simulink library "Lib_LongPRACH"  (R2023b)
settings: Solver=VariableStepAuto  StartTime=0.0  StopTime=10.0  RelTol=1e-3
values from neighbouring files (symbols this model uses):
  prach = waveconfig.PRACH.Config    [hNRPRACHWaveformGenerator.m]
undefined symbols (not defined in the file or in its folder): AdvDSPBChannelOutDisplay, AdvDSPBDMemDisplay, AdvDSPBInDisplay, AdvDSPBOutDisplay, dpoly, dspba, dspba_ChannelInVis, dspba_ChannelOutVis, dspba_internal_get_channel_ports, evalAionMaskParam, latency, latencyCorrection, NTxAnts, primtype, UseDontCare, value
libraries: DSPBAPrim x553, DSPBABase x32, DSPBAFilters x24, DSPBAControl x18, DSPBAModelBus x8, DSPBAWaveformSynth x4, DspbAdvFftLibrary x2, DSPBAUtilities x2
(part 5 of 8)

== system Lib_LongPRACH/prach_wrap/SYM_SELECT/Zero_insertion ==
  valid_in : Inport
  chin : Inport  Port=2
  datain : Inport  Port=3
  To Workspace1 : ToWorkspace  VariableName=zeropad_front_ch  SampleTime=-1
  To Workspace2 : ToWorkspace  VariableName=zeropad_front_data  SampleTime=-1
  To Workspace7 : ToWorkspace  VariableName=zeropad_front_v  SampleTime=-1
  Zeropad_front : Subsystem
  Zeropad_rear : Subsystem
  valid_out : Outport
  "chout " : Outport  Port=2
  dataout : Outport  Port=3
  wires:
  valid_in/1 -> Zeropad_front/1(valid_in)
  datain/1 -> Zeropad_front/3(datain)
  chin/1 -> Zeropad_front/2(chin)
  Zeropad_front/1(valid_out) -> To Workspace7/1, Zeropad_rear/1(valid_in)
  Zeropad_front/2("chout ") -> To Workspace1/1, Zeropad_rear/2(chin)
  Zeropad_front/3(dataout) -> To Workspace2/1, Zeropad_rear/3(datain)
  Zeropad_rear/1(valid_out) -> valid_out/1
  Zeropad_rear/2("chout ") -> "chout "/1
  Zeropad_rear/3(dataout) -> dataout/1

== system Lib_LongPRACH/Longprach_C_M_plane/LongPRACH_core/CP_REMOVAL/RemoveCP5 ==
  vin : Inport
  chin : Inport  Port=2
  din : Inport  Port=3
  cp_start : Inport  Port=4
  gt_end : Inport  Port=5
  filt_flush_en : Inport  Port=6
  And1 : DSPBAPrim/And  primtype=and  nInputs=3  nOutputs=1  omode=Inherit via internal rule  otype=sfix(16)  scale=2^-15  rndmethod=Unbiased  factor=1  satmethod=Symmetric  shift_vec=[0 1 2 -1]  value=0  inPortNames=[' '; ' '; ' '; ' '; ' '; ' '; ' '; ' '; ' '; ' '; ' '; ' '; ' '; ' '; ' '; ' '; ]  outPortNames=[' ']  dspbaimage=dspba_prim.svg  text=fprintf('&');  style=Optimised  visibilities=8+2  version=20211007
  And2 : DSPBAPrim/And  primtype=and  nInputs=3  nOutputs=1  omode=Inherit via internal rule  otype=sfix(16)  scale=2^-15  rndmethod=Unbiased  factor=1  satmethod=Symmetric  shift_vec=[0 1 2 -1]  value=0  inPortNames=[' '; ' '; ' '; ' '; ' '; ' '; ' '; ' '; ' '; ' '; ' '; ' '; ' '; ' '; ' '; ' '; ]  outPortNames=[' ']  dspbaimage=dspba_prim.svg  text=fprintf('&');  style=Optimised  visibilities=8+2  version=20211007
  ChannelIn : DSPBAPrim/ChannelIn  primtype=channelin  nInputs=dspba_internal_get_channel_ports(gcb)  nOutputs=dspba_internal_get_channel_ports(gcb)  omode=Inherit via internal rule  otype=sfix(16)  scale=2^-15  rndmethod=Unbiased  factor=1  satmethod=Symmetric  shift_vec=[0 1 2 -1]  value=4  inPortNames=['v'; 'c'; '0'; '1'; '2'; '3'; '4'; '5'; '6'; '7'; '8'; '9'; 'A'; 'B'; 'D'; 'E'; 'F'; 'G'; 'H'; 'I'; 'J'; 'K'; 'L'; 'M'; 'N'; 'O'; 'P'; 'Q'; 'R'; 'S'; 'T'; 'U'; 'W'; 'X'; 'Y'; 'Z']  outPortNames=['v'; 'c'; '0'; '1'; '2'; '3'; '4'; '5'; '6'; '7'; '8'; '9'; 'A'; 'B'; 'D'; 'E'; 'F'; 'G'; 'H'; 'I'; 'J'; 'K'; 'L'; 'M'; 'N'; 'O'; 'P'; 'Q'; 'R'; 'S'; 'T'; 'U'; 'W'; 'X'; 'Y'; 'Z']  dspbaimage=dspba_prim_channel_tall.svg  text=fprintf('In');  style=Optimised  dataSignals=4  foldingEnabled=off  channels=1  sampleRate=200  packetBeginPresent=off  packetBeginEnabled=off  visibilities=dspba_ChannelInVis(gcb)  latencyCorrection=0  scheduleOrigin=on  version=20211214
  ChannelOut : DSPBAPrim/ChannelOut  primtype=channelout  nInputs=dspba_internal_get_channel_ports(gcb)  nOutputs=dspba_internal_get_channel_ports(gcb)  omode=Inherit via internal rule  otype=sfix(16)  scale=2^-15  rndmethod=Unbiased  factor=1  satmethod=Symmetric  shift_vec=[0 1 2 -1]  value=3  inPortNames=['v'; 'c'; '0'; '1'; '2'; '3'; '4'; '5'; '6'; '7'; '8'; '9'; 'A'; 'B'; 'D'; 'E'; 'F'; 'G'; 'H'; 'I'; 'J'; 'K'; 'L'; 'M'; 'N'; 'O'; 'P'; 'Q'; 'R'; 'S'; 'T'; 'U'; 'W'; 'X'; 'Y'; 'Z']  outPortNames=['v'; 'c'; '0'; '1'; '2'; '3'; '4'; '5'; '6'; '7'; '8'; '9'; 'A'; 'B'; 'D'; 'E'; 'F'; 'G'; 'H'; 'I'; 'J'; 'K'; 'L'; 'M'; 'N'; 'O'; 'P'; 'Q'; 'R'; 'S'; 'T'; 'U'; 'W'; 'X'; 'Y'; 'Z']  dspbaimage=dspba_prim_channel_tall.svg  text=fprintf('Out%s', AdvDSPBChannelOutDisplay(latency));  style=Optimised  dataSignals=3  foldingEnabled=off  channels=1  sampleRate=200  packetBeginPresent=off  packetBeginEnabled=off  visibilities=dspba_ChannelOutVis(gcb)  latency=3  latencyCorrection=0  version=20211214
  CmpGE_cpstart : DSPBAPrim/CmpGE  primtype=cmpgte  nInputs=2  nOutputs=1  omode=boolean  otype=sfix(16)  scale=2^-15  rndmethod=Unbiased  factor=1  satmethod=Symmetric  shift_vec=[0 1 2 -1]  value=0  inPortNames=['a'; 'b';]  outPortNames=[' ']  dspbaimage=dspba_prim.svg  text=fprintf('a>=b');  style=Optimised  visibilities=0  advOptions=[]  version=20211007
  CmpGE_cpstart1 : DSPBAPrim/CmpGE  primtype=cmpgte  nInputs=2  nOutputs=1  omode=boolean  otype=sfix(16)  scale=2^-15  rndmethod=Unbiased  factor=1  satmethod=Symmetric  shift_vec=[0 1 2 -1]  value=0  inPortNames=['a'; 'b';]  outPortNames=[' ']  dspbaimage=dspba_prim.svg  text=fprintf('a>=b');  style=Optimised  visibilities=0  advOptions=[]  version=20211007
  CmpLT_gaurdtime : DSPBAPrim/CmpLT  primtype=cmplt  nInputs=2  nOutputs=1  omode=boolean  otype=sfix(16)  scale=2^-15  rndmethod=Unbiased  factor=1  satmethod=Symmetric  shift_vec=[0 1 2 -1]  value=0  inPortNames=['a'; 'b';]  outPortNames=[' ']  dspbaimage=dspba_prim.svg  text=fprintf('a<b');  style=Optimised  visibilities=0  advOptions=[]  version=20211007
  CmpLT_gaurdtime1 : DSPBAPrim/CmpLT  primtype=cmplt  nInputs=2  nOutputs=1  omode=boolean  otype=sfix(16)  scale=2^-15  rndmethod=Unbiased  factor=1  satmethod=Symmetric  shift_vec=[0 1 2 -1]  value=0  inPortNames=['a'; 'b';]  outPortNames=[' ']  dspbaimage=dspba_prim.svg  text=fprintf('a<b');  style=Optimised  visibilities=0  advOptions=[]  version=20211007
  Const : DSPBAPrim/Const  primtype=const  nInputs=0  nOutputs=1  omode=Inherit via internal rule  otype=sfix(16)  scale=2^-15  rndmethod=Unbiased  factor=1  satmethod=Symmetric  shift_vec=[0 1 2 -1]  value=filt_flush_start  inPortNames=['+'; '+';]  outPortNames=[' ']  dspbaimage=dspba_prim.svg  text=fprintf('%s', num2str(value));  style=Optimised  visibilities=8 + 1024 + 2^18 + 2^20  floatPrecision=float32_m23  warnSaturation=on  version=20211007  SampleTime=inf
  Const1 : DSPBAPrim/Const  primtype=const  nInputs=0  nOutputs=1  omode=Inherit via internal rule  otype=sfix(16)  scale=2^-15  rndmethod=Unbiased  factor=1  satmethod=Symmetric  shift_vec=[0 1 2 -1]  value=filt_flush_end  inPortNames=['+'; '+';]  outPortNames=[' ']  dspbaimage=dspba_prim.svg  text=fprintf('%s', num2str(value));  style=Optimised  visibilities=8 + 1024 + 2^18 + 2^20  floatPrecision=float32_m23  warnSaturation=on  version=20211007  SampleTime=inf
  Convert : DSPBAPrim/Convert  primtype=convert  nInputs=1  nOutputs=1  omode=boolean  otype=sfix(16)  scale=2^-15  rndmethod=Unbiased  factor=1  satmethod=None  shift_vec=[0 1 2 -1]  value=round([0:255]/17)  inPortNames=[' '; ' ';]  outPortNames=[' '; 'c']  dspbaimage=dspba_prim_wide.svg  text=fprintf('convert');  style=Optimised  visibilities=8+64+256+2^17  clipdetect=off  floatPrecision=float32_m23  advOptions=[]  version=20211007
  Counter : DSPBAPrim/Counter  primtype=counter  nInputs=1  nOutputs=1  omode=Inherit via internal rule  otype=ufix(16)  scale=2^-0  rndmethod=Unbiased  factor=1  satmethod=Symmetric  shift_vec=[0 1 2 -1]  value=[prach.symPeriod_dec-1 prach.symPeriod_dec 1]  inPortNames=[' '; ' ';]  outPortNames=[' ']  dspbaimage=dspba_prim.svg  text=fprintf('counter\n[%d %d %d]', value(1), value(2), value(3));  style=Optimised  visibilities=8 + 1024  version=20211007
  SynthesisInfo : DSPBAPrim/SynthesisInfo  primtype=synthinfo  nInputs=0  nOutputs=0  omode=Inherit via internal rule  otype=sfix(16)  scale=2^-15  rndmethod=Truncate  factor=1  satmethod=Symmetric  shift_vec=[0 1 2 -1]  value=99  inPortNames=[' '; ' ';]  outPortNames=[' ']  dspbaimage=dspba_prim_ctrl.jpg  text=fprintf('Style=%s', style);  style=Scheduled  visibilities=2^17+2^18+2^19+2^20+2^21+2^22+2^23+2^24  constraintPair=None  constraintRelation=>  constraintLimit=6  modelRefSign=+  modelRef=''  showSchedule=off  simulationMode=Use Global Value  resetMinimization=Conditional - On for ChannelIn/Out only  version=20220106
  input2 : Scope  NumInputPorts=3
  syncgen : Subsystem
  vout : Outport  VectorParamsAs1DForOutWhenUnconnected=off
  cout : Outport  Port=2  VectorParamsAs1DForOutWhenUnconnected=off
  dout : Outport  Port=3  VectorParamsAs1DForOutWhenUnconnected=off
  filt_flush : Outport  Port=4  VectorParamsAs1DForOutWhenUnconnected=off
  sync_out : Outport  Port=5
  wires:
  ChannelIn/5 -> CmpLT_gaurdtime/2
  ChannelIn/4 -> CmpGE_cpstart/2
  cp_start/1 -> ChannelIn/4
  gt_end/1 -> ChannelIn/5
  ChannelIn/3 -> ChannelOut/3
  CmpLT_gaurdtime/1 -> And1/3
  CmpGE_cpstart/1 -> And1/2
  vin/1 -> ChannelIn/1
  chin/1 -> ChannelIn/2
  din/1 -> ChannelIn/3
  ChannelOut/3 -> dout/1
  ChannelOut/2 -> cout/1
  ChannelOut/1 -> vout/1
  ChannelIn/1 -> Counter/1, input2/1, And1/1
  ChannelIn/2 -> ChannelOut/2
  And1/1 -> input2/3, ChannelOut/1
  CmpGE_cpstart1/1 -> And2/1
  Counter/1 -> CmpLT_gaurdtime1/1, CmpGE_cpstart1/1, syncgen/1(In1), CmpGE_cpstart/1, input2/2, CmpLT_gaurdtime/1
  CmpLT_gaurdtime1/1 -> And2/2
  And2/1 -> ChannelOut/4
  ChannelOut/4 -> filt_flush/1
  ChannelIn/6 -> Convert/1
  Convert/1 -> And2/3
  Const/1 -> CmpGE_cpstart1/2
  Const1/1 -> CmpLT_gaurdtime1/2
  filt_flush_en/1 -> ChannelIn/6
  syncgen/1(q) -> ChannelOut/5
  ChannelOut/5 -> sync_out/1

== system Lib_LongPRACH/Longprach_C_M_plane/LongPRACH_core/DECIMATION1/Stage1 ==
  data_in : Inport
  valid_in : Inport  Port=2
  ch_in : Inport  Port=3
  flush_en : Inport  Port=4
  Filt_DEC_by_3_stage1 : Subsystem
  filt_flush_in : Subsystem
  data_out : Outport
  valid_out : Outport  Port=2
  ch_out : Outport  Port=3
  wires:
  Filt_DEC_by_3_stage1/3(cout) -> ch_out/1
  Filt_DEC_by_3_stage1/2(vout) -> valid_out/1
  data_in/1 -> filt_flush_in/1(data_in)
  filt_flush_in/1(data_out) -> Filt_DEC_by_3_stage1/1(din)
  Filt_DEC_by_3_stage1/1(dout) -> data_out/1
  filt_flush_in/2(valid_out) -> Filt_DEC_by_3_stage1/2(vin)
  filt_flush_in/3(ch_out) -> Filt_DEC_by_3_stage1/3(cin)
  flush_en/1 -> filt_flush_in/4(flush_en)
  valid_in/1 -> filt_flush_in/2(valid_in)
  ch_in/1 -> filt_flush_in/3(ch_in)

== system Lib_LongPRACH/Longprach_C_M_plane/LongPRACH_core/DECIMATION1/Stage2 ==
  data_in : Inport
  valid_in : Inport  Port=2
  ch_in : Inport  Port=3
  Filt_DEC_by_2_stage2 : Subsystem
  data_out : Outport
  valid_out : Outport  Port=2
  ch_out : Outport  Port=3
  wires:
  data_in/1 -> Filt_DEC_by_2_stage2/1(din)
  valid_in/1 -> Filt_DEC_by_2_stage2/2(vin)
  ch_in/1 -> Filt_DEC_by_2_stage2/3(cin)
  Filt_DEC_by_2_stage2/1(dout) -> data_out/1
  Filt_DEC_by_2_stage2/3(cout) -> ch_out/1
  Filt_DEC_by_2_stage2/2(vout) -> valid_out/1

== system Lib_LongPRACH/Longprach_C_M_plane/LongPRACH_core/DECIMATION1/Stage3 ==
  data_in : Inport
  valid_in : Inport  Port=2
  ch_in : Inport  Port=3
  Filt_DEC_by_2_stage3 : Subsystem
  data_out : Outport
  valid_out : Outport  Port=2
  ch_out : Outport  Port=3
  wires:
  valid_in/1 -> Filt_DEC_by_2_stage3/2(vin)
  Filt_DEC_by_2_stage3/1(dout) -> data_out/1
  Filt_DEC_by_2_stage3/3(cout) -> ch_out/1
  Filt_DEC_by_2_stage3/2(vout) -> valid_out/1
  ch_in/1 -> Filt_DEC_by_2_stage3/3(cin)
  data_in/1 -> Filt_DEC_by_2_stage3/1(din)

== system Lib_LongPRACH/Longprach_C_M_plane/LongPRACH_core/DECIMATION1/Stage5 ==
  data_in : Inport
  valid_in : Inport  Port=2
  ch_in : Inport  Port=3
  Filt_DEC_by_2_stage5 : Subsystem
  data_out : Outport
  valid_out : Outport  Port=2
  ch_out : Outport  Port=3
  wires:
  Filt_DEC_by_2_stage5/1(dout) -> data_out/1
  Filt_DEC_by_2_stage5/3(cout) -> ch_out/1
  data_in/1 -> Filt_DEC_by_2_stage5/1(din)
  Filt_DEC_by_2_stage5/2(vout) -> valid_out/1
  valid_in/1 -> Filt_DEC_by_2_stage5/2(vin)
  ch_in/1 -> Filt_DEC_by_2_stage5/3(cin)

== system Lib_LongPRACH/Longprach_C_M_plane/LongPRACH_core/DECIMATION1/Stage6 ==
  data_in : Inport
  valid_in : Inport  Port=2
  ch_in : Inport  Port=3
  flush_en : Inport  Port=4
  Filt_DEC_by_2_stage6 : Subsystem
  filt_flush_out : Subsystem
  data_out : Outport
  valid_out : Outport  Port=2
  ch_out : Outport  Port=3
  wires:
  data_in/1 -> Filt_DEC_by_2_stage6/1(din)
  valid_in/1 -> Filt_DEC_by_2_stage6/2(vin)
  ch_in/1 -> Filt_DEC_by_2_stage6/3(cin)
  filt_flush_out/1(data_out) -> data_out/1
  filt_flush_out/2(valid_out) -> valid_out/1
  filt_flush_out/3(ch_out) -> ch_out/1
  Filt_DEC_by_2_stage6/1(dout) -> filt_flush_out/1(data_in)
  Filt_DEC_by_2_stage6/2(vout) -> filt_flush_out/2(valid_in)
  Filt_DEC_by_2_stage6/3(cout) -> filt_flush_out/3(ch_in)
  flush_en/1 -> filt_flush_out/4(flush_en)

== system Lib_LongPRACH/Longprach_C_M_plane/LongPRACH_core/DECIMATION1/stage4 ==
  data_in : Inport
  valid_in : Inport  Port=2
  ch_in : Inport  Port=3
  Filt_DEC_by_2_stage4 : Subsystem
  data_out : Outport
  valid_out : Outport  Port=2
  ch_out : Outport  Port=3
  wires:
  Filt_DEC_by_2_stage4/3(cout) -> ch_out/1
  Filt_DEC_by_2_stage4/2(vout) -> valid_out/1
  data_in/1 -> Filt_DEC_by_2_stage4/1(din)
  ch_in/1 -> Filt_DEC_by_2_stage4/3(cin)
  Filt_DEC_by_2_stage4/1(dout) -> data_out/1
  valid_in/1 -> Filt_DEC_by_2_stage4/2(vin)

== system Lib_LongPRACH/Longprach_C_M_plane/LongPRACH_core/FFTShift/ChNoLatch ==
  valid1 : Inport
  din : Inport  Port=2
  valid2 : Inport  Port=3
  FIFO : DSPBAPrim/FIFO  primtype=fifo  nInputs=3  nOutputs=4  omode=Inherit via internal rule  otype=sfix(16)  scale=2^-15  rndmethod=Unbiased  factor=1  satmethod=Symmetric  shift_vec=[0 1 2 -1]  value=[32 4 16]  inPortNames=['w'; 'd'; 'r'; 'f']  outPortNames=['v'; 'q'; 't'; 'f']  dspbaimage=dspba_prim_tall.svg  text=fprintf('fifo');  style=Optimised  visibilities=263168  version=20211007  user_sclr=off
  Terminator1 : Terminator
  Terminator2 : Terminator
  Terminator3 : Terminator
  risingedge : Subsystem
  risingedge1 : Subsystem
  dout : Outport
  wires:
  din/1 -> FIFO/2
  valid1/1 -> risingedge/1(In2)
  FIFO/2 -> dout/1
  valid2/1 -> risingedge1/1(In2)
  risingedge/1(Out1) -> FIFO/1
  FIFO/4 -> Terminator2/1
  risingedge1/1(Out1) -> FIFO/3
  FIFO/1 -> Terminator3/1
  FIFO/3 -> Terminator1/1

== system Lib_LongPRACH/Longprach_C_M_plane/LongPRACH_core/FFTShift/Mem_rd_wr ==
  valid : Inport
  Mem_rd_control : Subsystem
  Mem_wr_control : Subsystem
  Wr_addr_final : Outport
  We : Outport  Port=2
  rd_addr_final : Outport  Port=3
  rd_validout : Outport  Port=4
  wba : Outport  Port=5
  wires:
  Mem_rd_control/2(validout) -> rd_validout/1
  Mem_rd_control/1(rd_addr_final) -> rd_addr_final/1
  Mem_wr_control/3(wba) -> Mem_rd_control/1(wba), wba/1
  Mem_wr_control/2(we) -> We/1
  Mem_wr_control/1(wr_addr_final) -> Wr_addr_final/1
  valid/1 -> Mem_wr_control/1(valid)

== system Lib_LongPRACH/Longprach_C_M_plane/LongPRACH_core/FFTShift/Subsystem ==
  toggleline : Inport
  d : Inport  Port=2
  SampleDelay : DSPBAPrim/SampleDelay  primtype=sampdelay  nInputs=1  nOutputs=1  omode=Inherit via internal rule  otype=sfix(16)  scale=2^-15  rndmethod=Unbiased  factor=1  satmethod=Symmetric  shift_vec=[0 1 2 -1]  floatPrecision=float32_m23  value=1  inPortNames=[' '; ' ';]  outPortNames=[' ']  dspbaimage=dspba_prim.svg  text=dpoly(1, eye(1,value+1), 'z')  style=Optimised  visibilities=8 + 2^11 + 2^18 + 2^19  flexible=off  slackgroup=0  augmented=0  version=20211007  advOptions=[]
  Xor : DSPBAPrim/Xor  primtype=xor  nInputs=2  nOutputs=1  omode=Inherit via internal rule  otype=sfix(16)  scale=2^-15  rndmethod=Unbiased  factor=1  satmethod=Symmetric  shift_vec=[0 1 2 -1]  value=0  inPortNames=[' '; ' '; ' '; ' '; ' '; ' '; ' '; ' '; ' '; ' '; ' '; ' '; ' '; ' '; ' '; ' '; ]  outPortNames=[' ']  dspbaimage=dspba_prim.svg  text=fprintf('^');  style=Optimised  visibilities=8+2  version=20211007
  latch_0L : DSPBAControl/latch_0L
  q : Outport
  wires:
  toggleline/1 -> Xor/2, SampleDelay/1
  d/1 -> latch_0L/2
  latch_0L/1 -> q/1
  Xor/1 -> latch_0L/1
  SampleDelay/1 -> Xor/1

== system Lib_LongPRACH/Longprach_C_M_plane/LongPRACH_core/S2B_FFT/S2B ==
  data_in : Inport
  data_valid : Inport  Port=2
  chin : Inport  Port=3
  resetin : Inport  Port=4
  ChannelIn : DSPBAPrim/ChannelIn  primtype=channelin  nInputs=dspba_internal_get_channel_ports(gcb)  nOutputs=dspba_internal_get_channel_ports(gcb)  omode=Inherit via internal rule  otype=sfix(16)  scale=2^-15  rndmethod=Unbiased  factor=1  satmethod=Symmetric  shift_vec=[0 1 2 -1]  value=2  inPortNames=['v'; 'c'; '0'; '1'; '2'; '3'; '4'; '5'; '6'; '7'; '8'; '9'; 'A'; 'B'; 'D'; 'E'; 'F'; 'G'; 'H'; 'I'; 'J'; 'K'; 'L'; 'M'; 'N'; 'O'; 'P'; 'Q'; 'R'; 'S'; 'T'; 'U'; 'W'; 'X'; 'Y'; 'Z']  outPortNames=['v'; 'c'; '0'; '1'; '2'; '3'; '4'; '5'; '6'; '7'; '8'; '9'; 'A'; 'B'; 'D'; 'E'; 'F'; 'G'; 'H'; 'I'; 'J'; 'K'; 'L'; 'M'; 'N'; 'O'; 'P'; 'Q'; 'R'; 'S'; 'T'; 'U'; 'W'; 'X'; 'Y'; 'Z']  dspbaimage=dspba_prim_channel_tall.svg  text=fprintf('In');  style=Optimised  dataSignals=2  foldingEnabled=off  channels=1  sampleRate=200  packetBeginPresent=off  packetBeginEnabled=off  visibilities=dspba_ChannelInVis(gcb)  latencyCorrection=0  scheduleOrigin=on  version=20211214
  ChannelOut : DSPBAPrim/ChannelOut  primtype=channelout  nInputs=dspba_internal_get_channel_ports(gcb)  nOutputs=dspba_internal_get_channel_ports(gcb)  omode=Inherit via internal rule  otype=sfix(16)  scale=2^-15  rndmethod=Unbiased  factor=1  satmethod=Symmetric  shift_vec=[0 1 2 -1]  value=1  inPortNames=['v'; 'c'; '0'; '1'; '2'; '3'; '4'; '5'; '6'; '7'; '8'; '9'; 'A'; 'B'; 'D'; 'E'; 'F'; 'G'; 'H'; 'I'; 'J'; 'K'; 'L'; 'M'; 'N'; 'O'; 'P'; 'Q'; 'R'; 'S'; 'T'; 'U'; 'W'; 'X'; 'Y'; 'Z']  outPortNames=['v'; 'c'; '0'; '1'; '2'; '3'; '4'; '5'; '6'; '7'; '8'; '9'; 'A'; 'B'; 'D'; 'E'; 'F'; 'G'; 'H'; 'I'; 'J'; 'K'; 'L'; 'M'; 'N'; 'O'; 'P'; 'Q'; 'R'; 'S'; 'T'; 'U'; 'W'; 'X'; 'Y'; 'Z']  dspbaimage=dspba_prim_channel_tall.svg  text=fprintf('Out%s', AdvDSPBChannelOutDisplay(latency));  style=Optimised  dataSignals=1  foldingEnabled=off  channels=1  sampleRate=200  packetBeginPresent=off  packetBeginEnabled=off  visibilities=dspba_ChannelOutVis(gcb)  latency=6  latencyCorrection=0  version=20211214
  DualMem : DSPBAPrim/DualMem  primtype=dualmem  nInputs=4  nOutputs=2  omode=Inherit via internal rule  otype=sfix(16)  scale=2^-15  rndmethod=Unbiased  factor=1  satmethod=Symmetric  shift_vec=[0 1 2 -1]  value=[zeros(1024*4*2, 1)]  inPortNames=['d1'; 'a1'; 'w1'; 'd2'; 'a2'; 'w2']  outPortNames=['q1'; 'q2']  dspbaimage=dspba_prim_tall.svg  text=fprintf('dmem%s',AdvDSPBDMemDisplay(UseDontCare));  style=Optimised  visibilities=8 + 1024 + 2^17 + 2^18  UseDontCare=on  TwinWritePorts=off  init=on  ProvideReadAccess=off  version=20211007
  S2B_control : Subsystem
  SynthesisInfo : DSPBAPrim/SynthesisInfo  primtype=synthinfo  nInputs=0  nOutputs=0  omode=Inherit via internal rule  otype=sfix(16)  scale=2^-15  rndmethod=Truncate  factor=1  satmethod=Symmetric  shift_vec=[0 1 2 -1]  value=99  inPortNames=[' '; ' ';]  outPortNames=[' ']  dspbaimage=dspba_prim_ctrl.jpg  text=fprintf('Style=%s', style);  style=Scheduled  visibilities=2^17+2^18+2^19+2^20+2^21+2^22+2^23+2^24  constraintPair=None  constraintRelation=>  constraintLimit=2  modelRefSign=+  modelRef=''  showSchedule=off  simulationMode=Use Global Value  resetMinimization=Conditional - On for ChannelIn/Out only  version=20220106
  Terminator : Terminator
  Terminator1 : Terminator
  data_out : Outport
  valid_out : Outport  Port=2
  ch_no : Outport  Port=3
  wires:
  ChannelOut/2 -> ch_no/1
  S2B_control/4(rd_validout) -> ChannelOut/1
  ChannelOut/1 -> valid_out/1
  DualMem/2 -> ChannelOut/3
  ChannelOut/3 -> data_out/1
  ChannelIn/2 -> Terminator1/1, S2B_control/2(ch_no_in)
  chin/1 -> ChannelIn/2
  data_valid/1 -> ChannelIn/1
  ChannelIn/1 -> S2B_control/1(valid)
  data_in/1 -> ChannelIn/3
  ChannelIn/3 -> DualMem/1
  S2B_control/5(ch_no) -> ChannelOut/2
  S2B_control/3(rd_addr_final) -> DualMem/4
  DualMem/1 -> Terminator/1
  S2B_control/1(Wr_addr_final) -> DualMem/2
  S2B_control/2(We) -> DualMem/3
  ChannelIn/4 -> S2B_control/3(resetin)
  resetin/1 -> ChannelIn/4

== system Lib_LongPRACH/Longprach_C_M_plane/LongPRACH_core/S2B_FFT/gain ==
  data_in : Inport
  data_valid : Inport  Port=2
  chin : Inport  Port=3
  gain : Inport  Port=4
  ChannelIn : DSPBAPrim/ChannelIn  primtype=channelin  nInputs=dspba_internal_get_channel_ports(gcb)  nOutputs=dspba_internal_get_channel_ports(gcb)  omode=Inherit via internal rule  otype=sfix(16)  scale=2^-15  rndmethod=Unbiased  factor=1  satmethod=Symmetric  shift_vec=[0 1 2 -1]  value=2  inPortNames=['v'; 'c'; '0'; '1'; '2'; '3'; '4'; '5'; '6'; '7'; '8'; '9'; 'A'; 'B'; 'D'; 'E'; 'F'; 'G'; 'H'; 'I'; 'J'; 'K'; 'L'; 'M'; 'N'; 'O'; 'P'; 'Q'; 'R'; 'S'; 'T'; 'U'; 'W'; 'X'; 'Y'; 'Z']  outPortNames=['v'; 'c'; '0'; '1'; '2'; '3'; '4'; '5'; '6'; '7'; '8'; '9'; 'A'; 'B'; 'D'; 'E'; 'F'; 'G'; 'H'; 'I'; 'J'; 'K'; 'L'; 'M'; 'N'; 'O'; 'P'; 'Q'; 'R'; 'S'; 'T'; 'U'; 'W'; 'X'; 'Y'; 'Z']  dspbaimage=dspba_prim_channel_tall.svg  text=fprintf('In');  style=Optimised  dataSignals=2  foldingEnabled=off  channels=1  sampleRate=200  packetBeginPresent=off  packetBeginEnabled=off  visibilities=dspba_ChannelInVis(gcb)  latencyCorrection=0  scheduleOrigin=on  version=20211214
  ChannelOut : DSPBAPrim/ChannelOut  primtype=channelout  nInputs=dspba_internal_get_channel_ports(gcb)  nOutputs=dspba_internal_get_channel_ports(gcb)  omode=Inherit via internal rule  otype=sfix(16)  scale=2^-15  rndmethod=Unbiased  factor=1  satmethod=Symmetric  shift_vec=[0 1 2 -1]  value=1  inPortNames=['v'; 'c'; '0'; '1'; '2'; '3'; '4'; '5'; '6'; '7'; '8'; '9'; 'A'; 'B'; 'D'; 'E'; 'F'; 'G'; 'H'; 'I'; 'J'; 'K'; 'L'; 'M'; 'N'; 'O'; 'P'; 'Q'; 'R'; 'S'; 'T'; 'U'; 'W'; 'X'; 'Y'; 'Z']  outPortNames=['v'; 'c'; '0'; '1'; '2'; '3'; '4'; '5'; '6'; '7'; '8'; '9'; 'A'; 'B'; 'D'; 'E'; 'F'; 'G'; 'H'; 'I'; 'J'; 'K'; 'L'; 'M'; 'N'; 'O'; 'P'; 'Q'; 'R'; 'S'; 'T'; 'U'; 'W'; 'X'; 'Y'; 'Z']  dspbaimage=dspba_prim_channel_tall.svg  text=fprintf('Out%s', AdvDSPBChannelOutDisplay(latency));  style=Optimised  dataSignals=1  foldingEnabled=off  channels=1  sampleRate=200  packetBeginPresent=off  packetBeginEnabled=off  visibilities=dspba_ChannelOutVis(gcb)  latency=6  latencyCorrection=0  version=20211214
  Convert : DSPBAPrim/Convert  primtype=convert  nInputs=1  nOutputs=1  omode=Specify via dialog  otype=sfix(16)  scale=2^-gain_out_frac  rndmethod=Unbiased  factor=1  satmethod=None  shift_vec=[0 1 2 -1]  value=round([0:255]/17)  inPortNames=[' '; ' ';]  outPortNames=[' '; 'c']  dspbaimage=dspba_prim_wide.svg  text=fprintf('convert');  style=Optimised  visibilities=8+64+256+2^17  clipdetect=off  floatPrecision=float32_m23  advOptions=[]  version=20211007
  Mult : DSPBAPrim/Mult  primtype=mult  nInputs=2  nOutputs=1  omode=Inherit via internal rule  otype=sfix(16)  scale=2^-15  rndmethod=Unbiased  factor=1  satmethod=Symmetric  shift_vec=[0 1 2 -1]  value=0  inPortNames=[' '; ' ';]  outPortNames=[' ']  dspbaimage=dspba_prim.svg  text=fprintf('X');  style=Optimised  visibilities=8+2^18+2^19  floatPrecision=float32_m23  floatRounding=correct  advOptions=[]  version=20211007
  SynthesisInfo : DSPBAPrim/SynthesisInfo  primtype=synthinfo  nInputs=0  nOutputs=0  omode=Inherit via internal rule  otype=sfix(16)  scale=2^-15  rndmethod=Truncate  factor=1  satmethod=Symmetric  shift_vec=[0 1 2 -1]  value=99  inPortNames=[' '; ' ';]  outPortNames=[' ']  dspbaimage=dspba_prim_ctrl.jpg  text=fprintf('Style=%s', style);  style=Scheduled  visibilities=2^17+2^18+2^19+2^20+2^21+2^22+2^23+2^24  constraintPair=None  constraintRelation=>  constraintLimit=2  modelRefSign=+  modelRef=''  showSchedule=off  simulationMode=Use Global Value  resetMinimization=Conditional - On for ChannelIn/Out only  version=20220106
  data_out : Outport
  valid_out : Outport  Port=2
  ch_no : Outport  Port=3
  wires:
  ChannelOut/2 -> ch_no/1
  ChannelOut/1 -> valid_out/1
  ChannelOut/3 -> data_out/1
  ChannelIn/2 -> ChannelOut/2
  chin/1 -> ChannelIn/2
  data_valid/1 -> ChannelIn/1
  data_in/1 -> ChannelIn/3
  gain/1 -> ChannelIn/4
  ChannelIn/1 -> ChannelOut/1
  ChannelIn/3 -> Mult/1
  ChannelIn/4 -> Mult/2
  Mult/1 -> Convert/1
  Convert/1 -> ChannelOut/3

== system Lib_LongPRACH/Longprach_C_M_plane/LongPRACH_core/SYM_SELECT/Zero_insertion ==
  valid_in : Inport
  chin : Inport  Port=2
  datain : Inport  Port=3
  To Workspace1 : ToWorkspace  VariableName=zeropad_front_ch  SampleTime=-1
  To Workspace2 : ToWorkspace  VariableName=zeropad_front_data  SampleTime=-1
  To Workspace7 : ToWorkspace  VariableName=zeropad_front_v  SampleTime=-1
  Zeropad_front : Subsystem
  Zeropad_rear : Subsystem
  valid_out : Outport
  "chout " : Outport  Port=2
  dataout : Outport  Port=3
  wires:
  Zeropad_rear/3(dataout) -> dataout/1
  Zeropad_rear/2("chout ") -> "chout "/1
  Zeropad_rear/1(valid_out) -> valid_out/1
  Zeropad_front/3(dataout) -> Zeropad_rear/3(datain), To Workspace2/1
  Zeropad_front/2("chout ") -> Zeropad_rear/2(chin), To Workspace1/1
  Zeropad_front/1(valid_out) -> Zeropad_rear/1(valid_in), To Workspace7/1
  chin/1 -> Zeropad_front/2(chin)
  datain/1 -> Zeropad_front/3(datain)
  valid_in/1 -> Zeropad_front/1(valid_in)

== system Lib_LongPRACH/Longprach_C_M_plane/LongPRACH_core/Timeref_capture_fifo/rising_edge ==
  In1 : Inport
  And : DSPBAPrim/And  primtype=and  nInputs=2  nOutputs=1  omode=Inherit via internal rule  otype=sfix(16)  scale=2^-15  rndmethod=Unbiased  factor=1  satmethod=Symmetric  shift_vec=[0 1 2 -1]  value=0  inPortNames=[' '; ' '; ' '; ' '; ' '; ' '; ' '; ' '; ' '; ' '; ' '; ' '; ' '; ' '; ' '; ' '; ]  outPortNames=[' ']  dspbaimage=dspba_prim.svg  text=fprintf('&');  style=Optimised  visibilities=8+2  version=20211007
  Not : DSPBAPrim/Not  primtype=not  nInputs=1  nOutputs=1  omode=Inherit via internal rule  otype=sfix(16)  scale=2^-15  rndmethod=Unbiased  factor=1  satmethod=Symmetric  shift_vec=[0 1 2 -1]  value=0  inPortNames=[' '; ' ';]  outPortNames=[' ']  dspbaimage=dspba_prim.svg  text=fprintf('~');  style=Optimised  visibilities=8  version=20211007
  SampleDelay : DSPBAPrim/SampleDelay  primtype=sampdelay  nInputs=1  nOutputs=1  omode=Inherit via internal rule  otype=sfix(16)  scale=2^-15  rndmethod=Unbiased  factor=1  satmethod=Symmetric  shift_vec=[0 1 2 -1]  floatPrecision=float32_m23  value=1  inPortNames=[' '; ' ';]  outPortNames=[' ']  dspbaimage=dspba_prim.svg  text=dpoly(1, eye(1,value+1), 'z')  style=Optimised  visibilities=8 + 2^11 + 2^18 + 2^19  flexible=off  slackgroup=0  augmented=0  version=20211007  advOptions=[]
  Out1 : Outport
  wires:
  In1/1 -> And/1, SampleDelay/1
  SampleDelay/1 -> Not/1
  And/1 -> Out1/1
  Not/1 -> And/2

== system Lib_LongPRACH/Longprach_C_M_plane/LongPRACH_core/Timeref_capture_fifo/rising_edge1 ==
  In1 : Inport
  And : DSPBAPrim/And  primtype=and  nInputs=2  nOutputs=1  omode=Inherit via internal rule  otype=sfix(16)  scale=2^-15  rndmethod=Unbiased  factor=1  satmethod=Symmetric  shift_vec=[0 1 2 -1]  value=0  inPortNames=[' '; ' '; ' '; ' '; ' '; ' '; ' '; ' '; ' '; ' '; ' '; ' '; ' '; ' '; ' '; ' '; ]  outPortNames=[' ']  dspbaimage=dspba_prim.svg  text=fprintf('&');  style=Optimised  visibilities=8+2  version=20211007
  Not : DSPBAPrim/Not  primtype=not  nInputs=1  nOutputs=1  omode=Inherit via internal rule  otype=sfix(16)  scale=2^-15  rndmethod=Unbiased  factor=1  satmethod=Symmetric  shift_vec=[0 1 2 -1]  value=0  inPortNames=[' '; ' ';]  outPortNames=[' ']  dspbaimage=dspba_prim.svg  text=fprintf('~');  style=Optimised  visibilities=8  version=20211007
  SampleDelay : DSPBAPrim/SampleDelay  primtype=sampdelay  nInputs=1  nOutputs=1  omode=Inherit via internal rule  otype=sfix(16)  scale=2^-15  rndmethod=Unbiased  factor=1  satmethod=Symmetric  shift_vec=[0 1 2 -1]  floatPrecision=float32_m23  value=1  inPortNames=[' '; ' ';]  outPortNames=[' ']  dspbaimage=dspba_prim.svg  text=dpoly(1, eye(1,value+1), 'z')  style=Optimised  visibilities=8 + 2^11 + 2^18 + 2^19  flexible=off  slackgroup=0  augmented=0  version=20211007  advOptions=[]
  Out1 : Outport
  wires:
  In1/1 -> And/1, SampleDelay/1
  SampleDelay/1 -> Not/1
  And/1 -> Out1/1
  Not/1 -> And/2

== system Lib_LongPRACH/Longprach_C_M_plane/MUX_ConfigId/DelayValid/Delayed_valid_gen ==
  Validin : Inport
  SubFN_Change : Inport  Port=2
  start_sym : Inport  Port=3
  CmpEQ4 : DSPBAPrim/CmpEQ  primtype=cmpeq  nInputs=2  nOutputs=1  omode=boolean  otype=sfix(16)  scale=2^-15  rndmethod=Unbiased  factor=1  satmethod=Symmetric  shift_vec=[0 1 2 -1]  value=0  inPortNames=[' '; ' ';]  outPortNames=[' ']  dspbaimage=dspba_prim.svg  text=fprintf('==');  style=Optimised  visibilities=0  advOptions=[]  version=20211007
  Const3 : DSPBAPrim/Const  primtype=const  nInputs=0  nOutputs=1  omode=boolean  otype=sfix(16)  scale=2^-15  rndmethod=Unbiased  factor=1  satmethod=Symmetric  shift_vec=[0 1 2 -1]  value=1  inPortNames=['+'; '+';]  outPortNames=[' ']  dspbaimage=dspba_prim.svg  text=fprintf('%s', num2str(value));  style=Optimised  visibilities=8 + 1024 + 2^18 + 2^20  floatPrecision=float32_m23  warnSaturation=on  version=20211007  SampleTime=inf
  Const4 : DSPBAPrim/Const  primtype=const  nInputs=0  nOutputs=1  omode=Inherit via internal rule  otype=sfix(16)  scale=2^-15  rndmethod=Unbiased  factor=1  satmethod=Symmetric  shift_vec=[0 1 2 -1]  value=Delay_Valid_by  inPortNames=['+'; '+';]  outPortNames=[' ']  dspbaimage=dspba_prim.svg  text=fprintf('%s', num2str(value));  style=Optimised  visibilities=8 + 1024 + 2^18 + 2^20  floatPrecision=float32_m23  warnSaturation=on  version=20211007  SampleTime=inf
  Const5 : DSPBAPrim/Const  primtype=const  nInputs=0  nOutputs=1  omode=Inherit via internal rule  otype=sfix(16)  scale=2^-15  rndmethod=Unbiased  factor=1  satmethod=Symmetric  shift_vec=[0 1 2 -1]  value=Delayed_Valid_len  inPortNames=['+'; '+';]  outPortNames=[' ']  dspbaimage=dspba_prim.svg  text=fprintf('%s', num2str(value));  style=Optimised  visibilities=8 + 1024 + 2^18 + 2^20  floatPrecision=float32_m23  warnSaturation=on  version=20211007  SampleTime=inf
  Const6 : DSPBAPrim/Const  primtype=const  nInputs=0  nOutputs=1  omode=Inherit via internal rule  otype=sfix(16)  scale=2^-15  rndmethod=Unbiased  factor=1  satmethod=Symmetric  shift_vec=[0 1 2 -1]  value=8  inPortNames=['+'; '+';]  outPortNames=[' ']  dspbaimage=dspba_prim.svg  text=fprintf('%s', num2str(value));  style=Optimised  visibilities=8 + 1024 + 2^18 + 2^20  floatPrecision=float32_m23  warnSaturation=on  version=20211007  SampleTime=inf
  Loop : DSPBAPrim/Loop  primtype=loop  nInputs=3  nOutputs=4  omode=Inherit via internal rule  otype=sfix(16)  scale=2^-15  rndmethod=Unbiased  factor=1  satmethod=Symmetric  shift_vec=[0 1 2 -1]  value=[zeros(16, 1)]  inPortNames=['g'; 'c'; 'e']  outPortNames=['v'; 'q'; 'f'; 'l']  dspbaimage=dspba_prim_tall.svg  text=fprintf('loop');  style=Optimised  visibilities=0  version=20211007
  Loop1 : DSPBAPrim/Loop  primtype=loop  nInputs=3  nOutputs=4  omode=Inherit via internal rule  otype=sfix(16)  scale=2^-15  rndmethod=Unbiased  factor=1  satmethod=Symmetric  shift_vec=[0 1 2 -1]  value=[zeros(16, 1)]  inPortNames=['g'; 'c'; 'e']  outPortNames=['v'; 'q'; 'f'; 'l']  dspbaimage=dspba_prim_tall.svg  text=fprintf('loop');  style=Optimised  visibilities=0  version=20211007
  Mux : DSPBAPrim/Mux  primtype=mux  nInputs=evalAionMaskParam(gcb,'value',1)+1  nOutputs=1  omode=Inherit via internal rule  otype=sfix(16)  scale=2^-15  rndmethod=Unbiased  factor=1  satmethod=Symmetric  shift_vec=[0 1 2 -1]  value=2  inPortNames=['s '; 'd0'; 'd1'; 'd2'; 'd3'; 'd4'; 'd5'; 'd6'; 'd7'; 'd8'; 'd9';]  outPortNames=[' ']  dspbaimage=dspba_prim_tall.svg  text=fprintf('%s', primtype);  style=Optimised  visibilities=1032  version=20211007
  SampleDelay : DSPBAPrim/SampleDelay  primtype=sampdelay  nInputs=1  nOutputs=1  omode=Inherit via internal rule  otype=sfix(16)  scale=2^-15  rndmethod=Unbiased  factor=1  satmethod=Symmetric  shift_vec=[0 1 2 -1]  floatPrecision=float32_m23  value=1  inPortNames=[' '; ' ';]  outPortNames=[' ']  dspbaimage=dspba_prim.svg  text=dpoly(1, eye(1,value+1), 'z')  style=Optimised  visibilities=8 + 2^11 + 2^18 + 2^19  flexible=off  slackgroup=0  augmented=0  version=20211007  advOptions=[]
  delay_valid : DSPBAPrim/And  primtype=and  nInputs=2  nOutputs=1  omode=Inherit via internal rule  otype=sfix(16)  scale=2^-15  rndmethod=Unbiased  factor=1  satmethod=Symmetric  shift_vec=[0 1 2 -1]  value=0  inPortNames=[' '; ' '; ' '; ' '; ' '; ' '; ' '; ' '; ' '; ' '; ' '; ' '; ' '; ' '; ' '; ' '; ]  outPortNames=[' ']  dspbaimage=dspba_prim.svg  text=fprintf('&');  style=Optimised  visibilities=8+2  version=20211007
  Valid_out : Outport
  wires:
  Validin/1 -> delay_valid/1
  SubFN_Change/1 -> delay_valid/2
  Const3/1 -> Loop/3, Loop1/3
  Const4/1 -> Loop/2
  Loop1/1 -> Valid_out/1
  Const5/1 -> Loop1/2
  Loop/4 -> SampleDelay/1
  delay_valid/1 -> Loop/1, Mux/2
  CmpEQ4/1 -> Mux/1
  start_sym/1 -> CmpEQ4/1
  Const6/1 -> CmpEQ4/2
  Mux/1 -> Loop1/1
  SampleDelay/1 -> Mux/3

== system Lib_LongPRACH/Longprach_C_M_plane/MUX_ConfigId/DelayValid/SFN_change1 ==
  SubFN : Inport
  CmpNE : DSPBAPrim/CmpNE  primtype=cmpne  nInputs=2  nOutputs=1  omode=boolean  otype=sfix(16)  scale=2^-15  rndmethod=Unbiased  factor=1  satmethod=Symmetric  shift_vec=[0 1 2 -1]  value=0  inPortNames=[' '; ' ';]  outPortNames=[' ']  dspbaimage=dspba_prim.svg  text=fprintf('~=');  style=Optimised  visibilities=0  advOptions=[]  version=20211007
  SampleDelay : DSPBAPrim/SampleDelay  primtype=sampdelay  nInputs=1  nOutputs=1  omode=Inherit via internal rule  otype=sfix(16)  scale=2^-15  rndmethod=Unbiased  factor=1  satmethod=Symmetric  shift_vec=[0 1 2 -1]  floatPrecision=float32_m23  value=1  inPortNames=[' '; ' ';]  outPortNames=[' ']  dspbaimage=dspba_prim.svg  text=dpoly(1, eye(1,value+1), 'z')  style=Optimised  visibilities=8 + 2^11 + 2^18 + 2^19  flexible=off  slackgroup=0  augmented=0  version=20211007  advOptions=[]
  SubFN_Change : Outport
  wires:
  SampleDelay/1 -> CmpNE/2
  CmpNE/1 -> SubFN_Change/1
  SubFN/1 -> CmpNE/1, SampleDelay/1

== system Lib_LongPRACH/Longprach_C_M_plane/MUX_ConfigId/StartSymLatch_at_oth_SubFN/DefaultLatch1 ==
  e : Inport
  d : Inport  Port=2
  init : Inport  Port=3
  Mux : DSPBAPrim/Mux  primtype=mux  nInputs=evalAionMaskParam(gcb,'value',1)+1  nOutputs=1  omode=Inherit via internal rule  otype=ufix(21)  scale=0  rndmethod=Unbiased  factor=1  satmethod=Symmetric  shift_vec=[0 1 2 -1]  value=2  inPortNames=['s '; 'd0'; 'd1'; 'd2'; 'd3'; 'd4'; 'd5'; 'd6'; 'd7'; 'd8'; 'd9';]  outPortNames=[' ']  dspbaimage=dspba_prim_tall.svg  text=fprintf('%s', primtype);  style=Optimised  visibilities=1032  version=20211007
  Or : DSPBAPrim/Or  primtype=or  nInputs=2  nOutputs=1  omode=boolean  otype=sfix(16)  scale=2^-15  rndmethod=Unbiased  factor=1  satmethod=Symmetric  shift_vec=[0 1 2 -1]  value=0  inPortNames=[' '; ' '; ' '; ' '; ' '; ' '; ' '; ' '; ' '; ' '; ' '; ' '; ' '; ' '; ' '; ' '; ]  outPortNames=[' ']  dspbaimage=dspba_prim.svg  text=fprintf('|');  style=Optimised  visibilities=8+2  version=20211007
  SameDT : DSPBAControl/SameDT
  SampleDelay : DSPBAPrim/SampleDelay  primtype=sampdelay  nInputs=1  nOutputs=1  omode=Inherit via internal rule  otype=sfix(16)  scale=2^-15  rndmethod=Unbiased  factor=1  satmethod=Symmetric  shift_vec=[0 1 2 -1]  floatPrecision=float32_m23  value=1  inPortNames=[' '; ' ';]  outPortNames=[' ']  dspbaimage=dspba_prim.svg  text=dpoly(1, eye(1,value+1), 'z')  style=Optimised  visibilities=8 + 2^11 + 2^18 + 2^19  flexible=off  slackgroup=0  augmented=0  version=20211007  advOptions=[]
  latch_0L : DSPBAControl/latch_0L
  latchout : Outport
  wires:
  d/1 -> latch_0L/2
  latch_0L/1 -> SameDT/1, Mux/3
  init/1 -> Mux/2
  SampleDelay/1 -> Or/2
  e/1 -> Or/1, latch_0L/1
  Mux/1 -> latchout/1, SameDT/2
  Or/1 -> Mux/1, SampleDelay/1

== system Lib_LongPRACH/Longprach_C_M_plane/MUX_ConfigId/StartSymLatch_at_oth_SubFN/SFN_change ==
  SubFN : Inport
  CmpNE : DSPBAPrim/CmpNE  primtype=cmpne  nInputs=2  nOutputs=1  omode=boolean  otype=sfix(16)  scale=2^-15  rndmethod=Unbiased  factor=1  satmethod=Symmetric  shift_vec=[0 1 2 -1]  value=0  inPortNames=[' '; ' ';]  outPortNames=[' ']  dspbaimage=dspba_prim.svg  text=fprintf('~=');  style=Optimised  visibilities=0  advOptions=[]  version=20211007
  SampleDelay : DSPBAPrim/SampleDelay  primtype=sampdelay  nInputs=1  nOutputs=1  omode=Inherit via internal rule  otype=sfix(16)  scale=2^-15  rndmethod=Unbiased  factor=1  satmethod=Symmetric  shift_vec=[0 1 2 -1]  floatPrecision=float32_m23  value=1  inPortNames=[' '; ' ';]  outPortNames=[' ']  dspbaimage=dspba_prim.svg  text=dpoly(1, eye(1,value+1), 'z')  style=Optimised  visibilities=8 + 2^11 + 2^18 + 2^19  flexible=off  slackgroup=0  augmented=0  version=20211007  advOptions=[]
  Out1 : Outport
  wires:
  SampleDelay/1 -> CmpNE/2
  CmpNE/1 -> Out1/1
  SubFN/1 -> CmpNE/1, SampleDelay/1

== system Lib_LongPRACH/prach_wrap/FFTShift/ChNoLatch/risingedge ==
  In2 : Inport
  And : DSPBAPrim/And  primtype=and  nInputs=2  nOutputs=1  omode=Inherit via internal rule  otype=sfix(16)  scale=2^-15  rndmethod=Unbiased  factor=1  satmethod=Symmetric  shift_vec=[0 1 2 -1]  value=0  inPortNames=[' '; ' '; ' '; ' '; ' '; ' '; ' '; ' '; ' '; ' '; ' '; ' '; ' '; ' '; ' '; ' '; ]  outPortNames=[' ']  dspbaimage=dspba_prim.svg  text=fprintf('&');  style=Optimised  visibilities=8+2  version=20211007
  Not : DSPBAPrim/Not  primtype=not  nInputs=1  nOutputs=1  omode=Inherit via internal rule  otype=sfix(16)  scale=2^-15  rndmethod=Unbiased  factor=1  satmethod=Symmetric  shift_vec=[0 1 2 -1]  value=0  inPortNames=[' '; ' ';]  outPortNames=[' ']  dspbaimage=dspba_prim.svg  text=fprintf('~');  style=Optimised  visibilities=8  version=20211007
  SampleDelay : DSPBAPrim/SampleDelay  primtype=sampdelay  nInputs=1  nOutputs=1  omode=Inherit via internal rule  otype=sfix(16)  scale=2^-15  rndmethod=Unbiased  factor=1  satmethod=Symmetric  shift_vec=[0 1 2 -1]  floatPrecision=float32_m23  value=1  inPortNames=[' '; ' ';]  outPortNames=[' ']  dspbaimage=dspba_prim.svg  text=dpoly(1, eye(1,value+1), 'z')  style=Optimised  visibilities=8 + 2^11 + 2^18 + 2^19  flexible=off  slackgroup=0  augmented=0  version=20211007  advOptions=[]
  Out1 : Outport
  wires:
  Not/1 -> And/2
  SampleDelay/1 -> Not/1
  In2/1 -> SampleDelay/1, And/1
  And/1 -> Out1/1

== system Lib_LongPRACH/prach_wrap/FFTShift/ChNoLatch/risingedge1 ==
  In2 : Inport
  And : DSPBAPrim/And  primtype=and  nInputs=2  nOutputs=1  omode=Inherit via internal rule  otype=sfix(16)  scale=2^-15  rndmethod=Unbiased  factor=1  satmethod=Symmetric  shift_vec=[0 1 2 -1]  value=0  inPortNames=[' '; ' '; ' '; ' '; ' '; ' '; ' '; ' '; ' '; ' '; ' '; ' '; ' '; ' '; ' '; ' '; ]  outPortNames=[' ']  dspbaimage=dspba_prim.svg  text=fprintf('&');  style=Optimised  visibilities=8+2  version=20211007
  Not : DSPBAPrim/Not  primtype=not  nInputs=1  nOutputs=1  omode=Inherit via internal rule  otype=sfix(16)  scale=2^-15  rndmethod=Unbiased  factor=1  satmethod=Symmetric  shift_vec=[0 1 2 -1]  value=0  inPortNames=[' '; ' ';]  outPortNames=[' ']  dspbaimage=dspba_prim.svg  text=fprintf('~');  style=Optimised  visibilities=8  version=20211007
  SampleDelay : DSPBAPrim/SampleDelay  primtype=sampdelay  nInputs=1  nOutputs=1  omode=Inherit via internal rule  otype=sfix(16)  scale=2^-15  rndmethod=Unbiased  factor=1  satmethod=Symmetric  shift_vec=[0 1 2 -1]  floatPrecision=float32_m23  value=1  inPortNames=[' '; ' ';]  outPortNames=[' ']  dspbaimage=dspba_prim.svg  text=dpoly(1, eye(1,value+1), 'z')  style=Optimised  visibilities=8 + 2^11 + 2^18 + 2^19  flexible=off  slackgroup=0  augmented=0  version=20211007  advOptions=[]
  Out1 : Outport
  wires:
  Not/1 -> And/2
  SampleDelay/1 -> Not/1
  In2/1 -> SampleDelay/1, And/1
  And/1 -> Out1/1

== system Lib_LongPRACH/prach_wrap/FFTShift/Mem_rd_wr/Mem_rd_control ==
  wba : Inport
  BitCombine : DSPBAPrim/BitCombine  primtype=bitcombine  nInputs=2  nOutputs=1  omode=Inherit via internal rule  otype=sfix(16)  scale=2^-15  rndmethod=Unbiased  factor=1  satmethod=Symmetric  shift_vec=[0 1 2 -1]  value=0  inPortNames=['l'; 'h';]  outPortNames=[' ']  dspbaimage=dspba_prim.svg  text=fprintf('[h,l]');  style=Optimised  visibilities=8+2  version=20211007
  Const1 : DSPBAPrim/Const  primtype=const  nInputs=0  nOutputs=1  omode=boolean  otype=fixdt(0,2,0)  scale=0  rndmethod=Unbiased  factor=1  satmethod=Symmetric  shift_vec=[0 1 2 -1]  value=1  inPortNames=['+'; '+';]  outPortNames=[' ']  dspbaimage=dspba_prim.svg  text=fprintf('%s', num2str(value));  style=Optimised  visibilities=8 + 1024  floatPrecision=float32_m23  warnSaturation=on  version=20211007  SampleTime=inf
  Const2 : DSPBAPrim/Const  primtype=const  nInputs=0  nOutputs=1  omode=Inherit via internal rule  otype=fixdt(0,10,0)  scale=0  rndmethod=Unbiased  factor=1  satmethod=Symmetric  shift_vec=[0 1 2 -1]  value=1024  inPortNames=['+'; '+';]  outPortNames=[' ']  dspbaimage=dspba_prim.svg  text=fprintf('%s', num2str(value));  style=Optimised  visibilities=8 + 1024  floatPrecision=float32_m23  warnSaturation=on  version=20211007  SampleTime=inf
  Convert : DSPBAPrim/Convert  primtype=convert  nInputs=1  nOutputs=1  omode=Specify via dialog  otype=fixdt(0,10,0)  scale=0  rndmethod=Unbiased  factor=1  satmethod=None  shift_vec=[0 1 2 -1]  value=round([0:255]/17)  inPortNames=[' '; ' ';]  outPortNames=[' '; 'c']  dspbaimage=dspba_prim_wide.svg  text=fprintf('convert');  style=Optimised  visibilities=8+64+256+2^17  clipdetect=off  floatPrecision=float32_m23  advOptions=[]  version=20211007
  EdgeDetect : Subsystem
  FFT_shiftAddrMap : Subsystem
  Loop : DSPBAPrim/Loop  primtype=loop  nInputs=3  nOutputs=4  omode=Inherit via internal rule  otype=sfix(16)  scale=2^-15  rndmethod=Unbiased  factor=1  satmethod=Symmetric  shift_vec=[0 1 2 -1]  value=[zeros(16, 1)]  inPortNames=['g'; 'c'; 'e']  outPortNames=['v'; 'q'; 'f'; 'l']  dspbaimage=dspba_prim_tall.svg  text=fprintf('loop');  style=Optimised  visibilities=0  version=20211007
  Not : DSPBAPrim/Not  primtype=not  nInputs=1  nOutputs=1  omode=Inherit via internal rule  otype=sfix(16)  scale=2^-15  rndmethod=Unbiased  factor=1  satmethod=Symmetric  shift_vec=[0 1 2 -1]  value=0  inPortNames=[' '; ' ';]  outPortNames=[' ']  dspbaimage=dspba_prim.svg  text=fprintf('~');  style=Optimised  visibilities=8  version=20211007
  rd_addr_final : Outport
  validout : Outport  Port=2
  wires:
  Const1/1 -> Loop/3
  Const2/1 -> Loop/2
  wba/1 -> Not/1, EdgeDetect/1(In1)
  EdgeDetect/1(Out1) -> Loop/1
  BitCombine/1 -> rd_addr_final/1
  Not/1 -> BitCombine/2  "rba"
  Loop/1 -> validout/1
  FFT_shiftAddrMap/1(Out1) -> BitCombine/1
  Convert/1 -> FFT_shiftAddrMap/1(In1)
  Loop/2 -> Convert/1

== system Lib_LongPRACH/prach_wrap/FFTShift/Mem_rd_wr/Mem_wr_control ==
  valid : Inport
  Wr_addr_gen : Subsystem
  wr_addr_final : Outport
  we : Outport  Port=2
  wba : Outport  Port=3
  wires:
  valid/1 -> Wr_addr_gen/1(valid)
  Wr_addr_gen/2(wr_addr) -> wr_addr_final/1
  Wr_addr_gen/3(we) -> we/1
  Wr_addr_gen/1(wba) -> wba/1

== system Lib_LongPRACH/prach_wrap/S2B_FFT/S2B/S2B_control ==
  valid : Inport
  Mem_rd_control : Subsystem
  Mem_wr_control : Subsystem
  Wr_addr_final : Outport
  We : Outport  Port=2
  rd_addr_final : Outport  Port=3
  rd_validout : Outport  Port=4
  ch_no : Outport  Port=5
  wires:
  valid/1 -> Mem_wr_control/1(valid)
  Mem_wr_control/1(wr_addr_final) -> Wr_addr_final/1
  Mem_wr_control/2(we) -> We/1
  Mem_wr_control/3(wba) -> Mem_rd_control/1(wba)
  Mem_rd_control/1(rd_addr_final) -> rd_addr_final/1
  Mem_rd_control/2(validout) -> rd_validout/1
  Mem_rd_control/3(ch_no) -> ch_no/1

== system Lib_LongPRACH/prach_wrap/SYM_SELECT/Zero_insertion/Zeropad_front ==
  valid_in : Inport
  chin : Inport  Port=2
  datain : Inport  Port=3
  And : DSPBAPrim/And  primtype=and  nInputs=2  nOutputs=1  omode=Inherit via internal rule  otype=sfix(16)  scale=2^-15  rndmethod=Unbiased  factor=1  satmethod=Symmetric  shift_vec=[0 1 2 -1]  value=0  inPortNames=[' '; ' '; ' '; ' '; ' '; ' '; ' '; ' '; ' '; ' '; ' '; ' '; ' '; ' '; ' '; ' '; ]  outPortNames=[' ']  dspbaimage=dspba_prim.svg  text=fprintf('&');  style=Optimised  visibilities=8+2  version=20211007
  Const3 : DSPBAPrim/Const  primtype=const  nInputs=0  nOutputs=1  omode=Inherit via internal rule  otype=sfix(16)  scale=2^-15  rndmethod=Unbiased  factor=1  satmethod=Symmetric  shift_vec=[0 1 2 -1]  value=0  inPortNames=['+'; '+';]  outPortNames=[' ']  dspbaimage=dspba_prim.svg  text=fprintf('%s', num2str(value));  style=Optimised  visibilities=8 + 1024 + 2^18 + 2^20  floatPrecision=float32_m23  warnSaturation=on  version=20211007  SampleTime=inf
  Mux1 : DSPBAPrim/Mux  primtype=mux  nInputs=evalAionMaskParam(gcb,'value',1)+1  nOutputs=1  omode=Inherit via internal rule  otype=sfix(16)  scale=2^-15  rndmethod=Unbiased  factor=1  satmethod=Symmetric  shift_vec=[0 1 2 -1]  value=2  inPortNames=['s '; 'd0'; 'd1'; 'd2'; 'd3'; 'd4'; 'd5'; 'd6'; 'd7'; 'd8'; 'd9';]  outPortNames=[' ']  dspbaimage=dspba_prim_tall.svg  text=fprintf('%s', primtype);  style=Optimised  visibilities=1032  version=20211007
  Not : DSPBAPrim/Not  primtype=not  nInputs=1  nOutputs=1  omode=Inherit via internal rule  otype=sfix(16)  scale=2^-15  rndmethod=Unbiased  factor=1  satmethod=Symmetric  shift_vec=[0 1 2 -1]  value=0  inPortNames=[' '; ' ';]  outPortNames=[' ']  dspbaimage=dspba_prim.svg  text=fprintf('~');  style=Optimised  visibilities=8  version=20211007
  Or : DSPBAPrim/Or  primtype=or  nInputs=2  nOutputs=1  omode=Inherit via internal rule  otype=sfix(16)  scale=2^-15  rndmethod=Unbiased  factor=1  satmethod=Symmetric  shift_vec=[0 1 2 -1]  value=0  inPortNames=[' '; ' '; ' '; ' '; ' '; ' '; ' '; ' '; ' '; ' '; ' '; ' '; ' '; ' '; ' '; ' '; ]  outPortNames=[' ']  dspbaimage=dspba_prim.svg  text=fprintf('|');  style=Optimised  visibilities=8+2  version=20211007
  SampleDelay1 : DSPBAPrim/SampleDelay  primtype=sampdelay  nInputs=1  nOutputs=1  omode=Inherit via internal rule  otype=sfix(16)  scale=2^-15  rndmethod=Unbiased  factor=1  satmethod=Symmetric  shift_vec=[0 1 2 -1]  floatPrecision=float32_m23  value=ZeroPadFront  inPortNames=[' '; ' ';]  outPortNames=[' ']  dspbaimage=dspba_prim.svg  text=dpoly(1, eye(1,value+1), 'z')  style=Optimised  visibilities=8 + 2^11 + 2^18 + 2^19  flexible=off  slackgroup=0  augmented=0  version=20211007  advOptions=[]
  SampleDelay2 : DSPBAPrim/SampleDelay  primtype=sampdelay  nInputs=1  nOutputs=1  omode=Inherit via internal rule  otype=sfix(16)  scale=2^-15  rndmethod=Unbiased  factor=1  satmethod=Symmetric  shift_vec=[0 1 2 -1]  floatPrecision=float32_m23  value=ZeroPadFront  inPortNames=[' '; ' ';]  outPortNames=[' ']  dspbaimage=dspba_prim.svg  text=dpoly(1, eye(1,value+1), 'z')  style=Optimised  visibilities=8 + 2^11 + 2^18 + 2^19  flexible=off  slackgroup=0  augmented=0  version=20211007  advOptions=[]
  valid_out : Outport
  "chout " : Outport  Port=2
  dataout : Outport  Port=3
  wires:
  Const3/1 -> Mux1/3
  Mux1/1 -> dataout/1
  Not/1 -> And/2
  Or/1 -> valid_out/1
  datain/1 -> SampleDelay1/1
  SampleDelay1/1 -> Mux1/2
  chin/1 -> "chout "/1
  SampleDelay2/1 -> Not/1, Or/2
  valid_in/1 -> And/1, Or/1, SampleDelay2/1
  And/1 -> Mux1/1
